simulink model "V1"  (R2025b)
settings: Solver=VariableStepAuto  StartTime=0.0  StopTime=3600*9  RelTol=1e-3
model workspace (MAT data in the model file):
  COP = 3.9
  Delayfan = [30 1]
  P1 = 1.05
  P2 = 1.91
  P3 = 1.91
  P4 = 1.05
  Q_Cond = 4.361
  Q_Evap = 3.471
  T1 = 12
  T2 = 37.72
  T3 = 29.61
  T4 = 7.9
  T_Enviroment_C = 27.5
  T_Room_int_C = 28.6
  T_Tank_int_c = 30
  Wall_h_in = 12
  Wall_h_out = 38
  h1 = 522.3
  h2 = 528.6
  h3 = 253.4
  h4 = 253.4
  m_dot = 0.014
libraries: fl_lib x102, nesl_utility x62, SimscapeFluids_lib x31
(part 4 of 4)

== stateflow chart V1/Chart1 ==
  state Charge
    entry :Evap = 0;Comp=1;Cond=1;
    Pump = 1;V_R32 = -1
  state Off
    entry :Evap = 0;Comp=0;Cond=0;
    Pump = 1;
  state Valve
    entry :V_R32 =1;
  state OffPump
    entry :Evap = 0;Comp=0;Cond=0;
    Pump = 0;
  (default) -> Charge
  Valve -> Off : [T_tank <10]
  Charge -> Valve : [T_Tank <=10]
  Off -> OffPump : [T_tank <9]
  data: T_Tank input; Comp output; Cond output; Evap output; Pump output; V_R32 output; T_tank input

== stateflow chart V1/Chart2 ==
  state Charge
    entry :Evap = 0;Comp=1;Cond=1;
    Pump = 1;
    V_R32 = -1;
    V_main = -1;
    V_discharge =1;
  state ChangValve1
    entry :Evap = 0;Comp=0;Cond=0;
    Pump = 1;
    V_R32 = 1;
    V_main = -1;
    V_discharge =1;
  state Off
    entry :Evap = 0;Comp=0;Cond=0;
    Pump = 0;
    V_R32 = 1;
    V_main = -1;
    V_discharge =1;
  state ChangeValve2
    entry :Evap = 0;Comp=0;Cond=0;
    Pump = 0;
    V_R32 = 1;
    V_main = 1;
    V_discharge =-1;
  state Discharge
    entry :Evap = 0.3;Comp=0;Cond=0;
    Pump = 0.5;
  state AC
    entry :Evap = 0.9;Comp=1;Cond=1;
    Pump = 0;
    V_R32 = 1;
    V_main = 1;
    V_discharge =1;
  (default) -> Charge
  Charge -> ChangValve1 : [T_Tank <=8]
  ChangValve1 -> Off : [after(60,sec)]
  Off -> ChangeValve2 : [after(60,sec)]
  ChangeValve2 -> Discharge : [after(5,sec)]
  Discharge -> AC : [T_Tank>18]
  data: T_Tank input; Comp output; Cond output; Evap output; Pump output; V_R32 output; T_Room input; V_discharge output; V_main output
